simulink model "dop2"  (R2018b)
settings: Solver=ode45  StartTime=0.0  StopTime=100  RelTol=1e-3  EnableMultiTasking=on
settings Model: Creator=bukova.2018  LastModifiedBy=Warnet
settings DataIOCC: LimitDataPoints=on  SaveFormat=Array
settings OptimizationCC: LifeSpan=inf
settings DebuggingCC: SolverPrmCheckMsg=warning  LibraryContextMissingDiagnostic=none  SFUnexpectedBacktrackingDiag=warning  SFNoUnconditionalDefaultTransitionDiag=warning  SFExecutionAtInitializationDiag=none
settings HardwareCC: ProdBitPerPointer=32  ProdBitPerSizeT=32  ProdBitPerPtrDiffT=32  ProdLargestAtomicFloat=None  ProdIntDivRoundTo=Undefined  ProdEndianess=Unspecified  ProdWordSize=32  ProdHWDeviceType=32-bit Generic
settings ModelReferenceCC: PropagateSignalLabelsOutOfModel=off
settings SFSimCC: SimUseLocalCustomCode=off
settings RTWCC: RTWUseLocalCustomCode=off
settings CodeAppCC: StateflowObjectComments=on
settings GRTTargetCC: TargetLangStandard=C89/C90 (ANSI)  GeneratePreprocessorConditionals=Disable all
settings ConfigComp: CovMetricSettings=dw  CovHtmlReporting=on  CovSaveCumulativeToWorkspaceVar=on  CovSaveSingleToWorkspaceVar=on  CovExternalEMLEnable=off  CovSFcnEnable=off

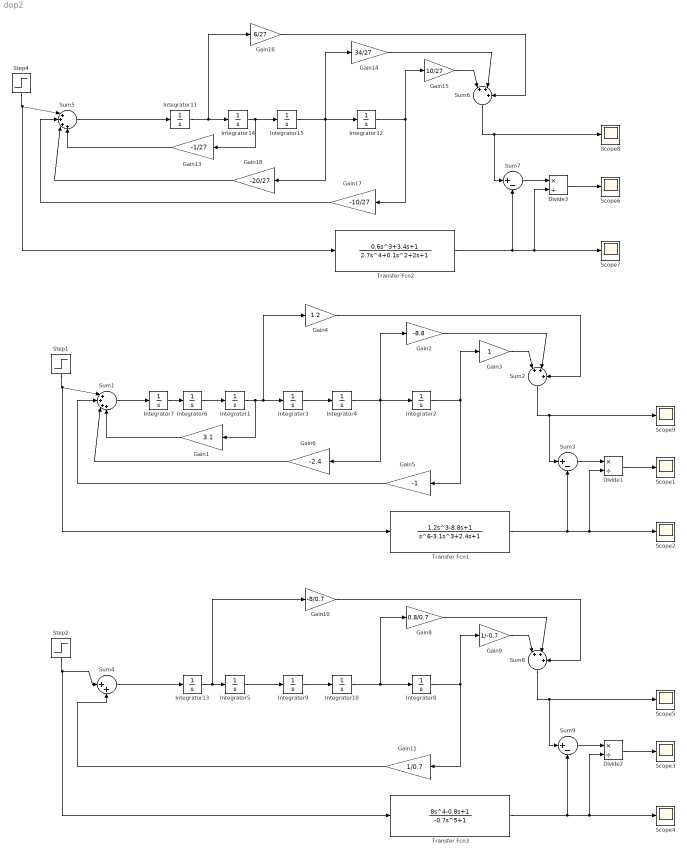
== system dop2 ==
  Divide1 : Product  Inputs=*/
  Divide2 : Product  Inputs=*/
  Divide3 : Product  Inputs=*/
  Gain1 : Gain  Gain=3.1
  Gain10 : Gain  Gain=-8/0.7
  Gain11 : Gain  Gain=1/0.7
  Gain13 : Gain  Gain=-1/27
  Gain14 : Gain  Gain=34/27
  Gain15 : Gain  Gain=10/27
  Gain16 : Gain  Gain=6/27
  Gain17 : Gain  Gain=-10/27
  Gain18 : Gain  Gain=-20/27
  Gain2 : Gain  Gain=-8.8
  Gain3 : Gain
  Gain4 : Gain  Gain=1.2
  Gain5 : Gain  Gain=-1
  Gain6 : Gain  Gain=-2.4
  Gain8 : Gain  Gain=0.8/0.7
  Gain9 : Gain  Gain=1/-0.7
  Integrator{1..15} (15 alike) : Integrator
  Scope{1..9} (9 alike) : Scope
  Step1 : Step  SampleTime=0
  Step2 : Step  SampleTime=0
  Step4 : Step  SampleTime=0
  Sum1 : Sum  Inputs=|++++
  Sum2 : Sum  Inputs=|+++
  Sum3 : Sum  Inputs=|+-
  Sum4 : Sum  Inputs=|++
  Sum5 : Sum  Inputs=|++++
  Sum6 : Sum  Inputs=|+++
  Sum7 : Sum  Inputs=|+-
  Sum8 : Sum  Inputs=|+++
  Sum9 : Sum  Inputs=|+-
  Transfer Fcn1 : TransferFcn  Numerator=[1.2 0 -8.8 1]  Denominator=[1 0 0 -3.1 0 2.4 1]
  Transfer Fcn2 : TransferFcn  Numerator=[0.6 0 3.4 1]  Denominator=[2.7 0 0.1 2 1 ]
  Transfer Fcn3 : TransferFcn  Numerator=[8 0 0 -0.8 1]  Denominator=[-0.7 0 0 0 0 1]
  wires:
  Integrator15/1 -> Gain14/1, Integrator12/1, Gain18/1
  Gain16/1 -> Sum6/3
  Integrator14/1 -> Integrator15/1, Gain13/1
  Gain17/1 -> Sum5/2
  Gain18/1 -> Sum5/3
  Gain15/1 -> Sum6/1
  Gain14/1 -> Sum6/2
  Integrator12/1 -> Gain15/1, Gain17/1
  Sum5/1 -> Integrator11/1
  Integrator11/1 -> Integrator14/1, Gain16/1
  Sum6/1 -> Scope8/1, Sum7/1
  Step4/1 -> Transfer Fcn2/1, Sum5/1
  Transfer Fcn2/1 -> Divide3/2, Scope7/1, Sum7/2
  Sum7/1 -> Divide3/1
  Divide3/1 -> Scope6/1
  Gain13/1 -> Sum5/4
  Divide1/1 -> Scope1/1
  Sum1/1 -> Integrator7/1
  Gain4/1 -> Sum2/3
  Integrator6/1 -> Integrator1/1
  Gain1/1 -> Sum1/4
  Integrator3/1 -> Integrator4/1
  Integrator7/1 -> Integrator6/1
  Integrator4/1 -> Gain2/1, Integrator2/1, Gain6/1
  Gain3/1 -> Sum2/1
  Integrator2/1 -> Gain3/1, Gain5/1
  Integrator1/1 -> Gain1/1, Integrator3/1, Gain4/1
  Gain2/1 -> Sum2/2
  Sum2/1 -> Scope9/1, Sum3/1
  Gain5/1 -> Sum1/2
  Gain6/1 -> Sum1/3
  Sum3/1 -> Divide1/1
  Transfer Fcn1/1 -> Divide1/2, Scope2/1, Sum3/2
  Step1/1 -> Transfer Fcn1/1, Sum1/1
  Gain8/1 -> Sum8/2
  Sum8/1 -> Scope5/1, Sum9/1
  Integrator13/1 -> Gain10/1, Integrator5/1
  Step2/1 -> Transfer Fcn3/1, Sum4/1
  Gain10/1 -> Sum8/3
  Transfer Fcn3/1 -> Divide2/2, Scope4/1, Sum9/2
  Integrator8/1 -> Gain9/1, Gain11/1
  Integrator5/1 -> Integrator9/1
  Divide2/1 -> Scope3/1
  Integrator10/1 -> Gain8/1, Integrator8/1
  Gain9/1 -> Sum8/1
  Gain11/1 -> Sum4/2
  Integrator9/1 -> Integrator10/1
  Sum4/1 -> Integrator13/1
  Sum9/1 -> Divide2/1
